simulink model "SISO_Simulation"  (R2020b)
settings: Solver=VariableStepAuto  StartTime=0.0  StopTime=10.0  RelTol=1e-3
PreLoadFcn:
  | loadSystemVariables
values from neighbouring files (symbols this model uses):
  Jl = 6.01e-5    (= 6.01e-05)    [loadSystemVariables.m]
  Jm = 996e-6    (= 0.000996)    [loadSystemVariables.m]
  Kb = (1/1000)*9.5493    (= 0.0095493)    [loadSystemVariables.m]
  Kf = 1    [loadSystemVariables.m]
  Kk = 1e4    (= 10000)    [loadSystemVariables.m]
  Km = 0.5    [loadSystemVariables.m]
  Kt = 18.16e-3    (= 0.01816)    [loadSystemVariables.m]
  Kv = 1000    [loadSystemVariables.m]
  L = series(P,G)    [SISO_phi.m]    (also in SISO_x.m; basicSISO_phi.m; basicSISO_x.m; basicSISO_y.m)
  R = 0.256    [loadSystemVariables.m]
libraries: uavalgslib x1
settings Model: Creator=Iftah  LastModifiedBy=Iftah

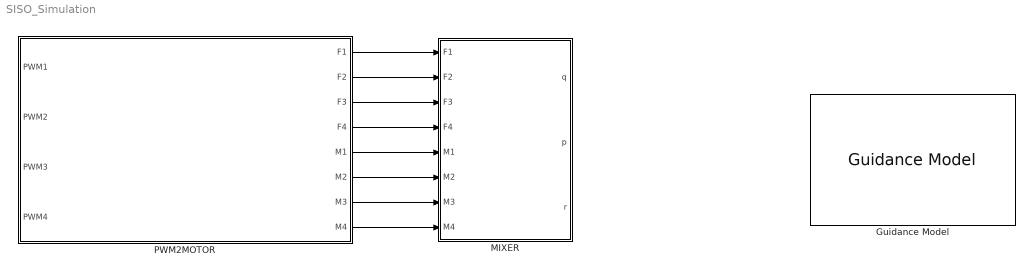
== system SISO_Simulation ==
  Guidance Model : uavalgslib/Guidance Model  ModelType=MultirotorGuidance  SpecifiedDataType=double  SimulateUsing=Interpreted execution  InitialWorldPositionMultirotor=[0; 0; 0]  InitialWorldVelocityMultirotor=[0; 0; 0]  InitialEulerZYXMultirotor=[0; 0; 0]  InitialBodyAngularRateRPYMultirotor=[0; 0; 0]  InitialThrustMultirotor=0  InitialNorthFixedWing=0  InitialEastFixedWing=0  InitialHeightFixedWing=0  InitialAirSpeedFixedWing=0  InitialHeadingAngleFixedWing=0  InitialFlightPathAngleFixedWing=0  InitialRollAngleFixedWing=0  InitialRollAngleRateFixedWing=0  PDRollMultirotor=[3402.97,116.67]  PDPitchMultirotor=[3402.97, 116.67]  PYawRateMultirotor=1950  PThrustMultirotor=3900  MassMultirotor=0.1  PHeightFixedWing=3.9  PHeadingAngleFixedWing=3.9  PFlightPathAngleFixedWing=39  PDRollFixedWing=[3402.97, 116.67]  PAirSpeedFixedWing=1  FlightPathAngleLimitsFixedWing=[-pi/2, pi/2]  StateBusName='MultirotorGuidanceStateBus'  ControlBusName='MultirotorGuidanceControlBus'  EnvironmentBusName='MultirotorGuidanceEnvironmentBus'  DataType=double
      settings: SourceProductBaseCode=UV
  MIXER : Subsystem
  PWM2MOTOR : Subsystem
  wires:
  PWM2MOTOR/1(F1) -> MIXER/1(F1)
  PWM2MOTOR/2(F2) -> MIXER/2(F2)
  PWM2MOTOR/3(F3) -> MIXER/3(F3)
  PWM2MOTOR/4(F4) -> MIXER/4(F4)
  PWM2MOTOR/5(M1) -> MIXER/5(M1)
  PWM2MOTOR/6(M2) -> MIXER/6(M2)
  PWM2MOTOR/7(M3) -> MIXER/7(M3)
  PWM2MOTOR/8(M4) -> MIXER/8(M4)

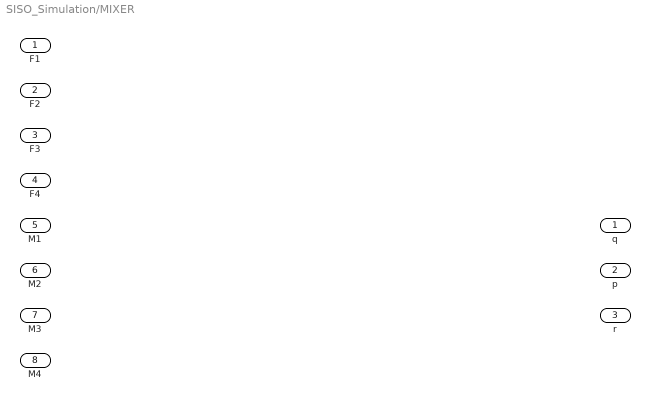
== system SISO_Simulation/MIXER ==
  F1 : Inport
  F2 : Inport  Port=2
  F3 : Inport  Port=3
  F4 : Inport  Port=4
  M1 : Inport  Port=5
  M2 : Inport  Port=6
  M3 : Inport  Port=7
  M4 : Inport  Port=8
  q : Outport
  p : Outport  Port=2
  r : Outport  Port=3

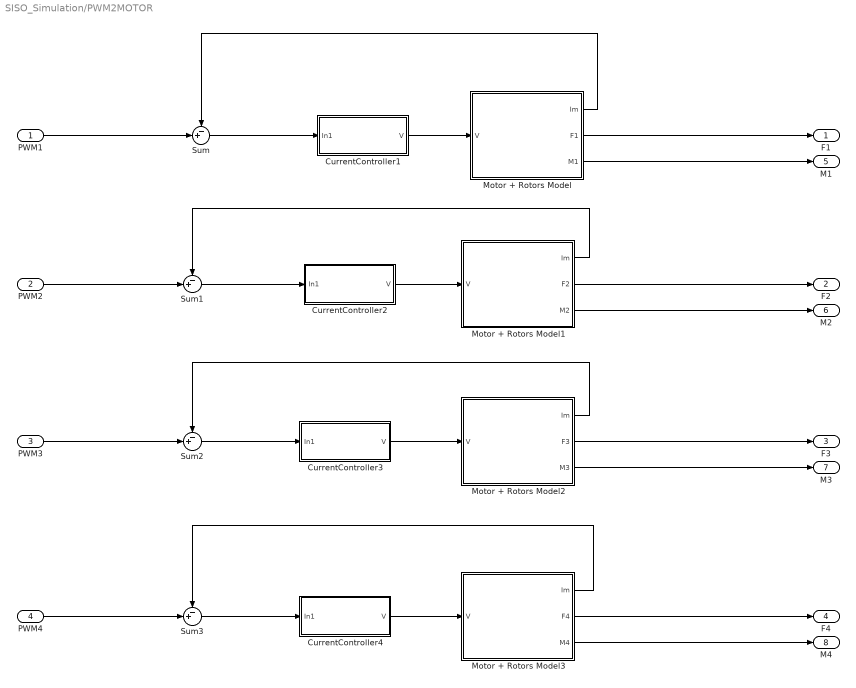
== system SISO_Simulation/PWM2MOTOR ==
  PWM1 : Inport
  PWM2 : Inport  Port=2
  PWM3 : Inport  Port=3
  PWM4 : Inport  Port=4
  CurrentController1 : Subsystem
  CurrentController2 : Subsystem
  CurrentController3 : Subsystem
  CurrentController4 : Subsystem
  Motor + Rotors Model : Subsystem
  Motor + Rotors Model1 : Subsystem
  Motor + Rotors Model2 : Subsystem
  Motor + Rotors Model3 : Subsystem
  Sum{,1..3} (4 alike) : Sum  Inputs=-+|
  F1 : Outport
  F2 : Outport  Port=2
  F3 : Outport  Port=3
  F4 : Outport  Port=4
  M1 : Outport  Port=5
  M2 : Outport  Port=6
  M3 : Outport  Port=7
  M4 : Outport  Port=8
  wires:
  Motor + Rotors Model/2(F1) -> F1/1
  Motor + Rotors Model/1(Im) -> Sum/1
  Motor + Rotors Model3/1(Im) -> Sum3/1
  Motor + Rotors Model1/3(M2) -> M2/1
  CurrentController3/1(V) -> Motor + Rotors Model2/1(V)
  Motor + Rotors Model1/2(F2) -> F2/1
  PWM1/1 -> Sum/2
  CurrentController1/1(V) -> Motor + Rotors Model/1(V)
  PWM3/1 -> Sum2/2
  Sum2/1 -> CurrentController3/1(In1)
  Motor + Rotors Model2/1(Im) -> Sum2/1
  Motor + Rotors Model3/2(F4) -> F4/1
  Sum/1 -> CurrentController1/1(In1)
  Motor + Rotors Model2/2(F3) -> F3/1
  Motor + Rotors Model/3(M1) -> M1/1
  CurrentController2/1(V) -> Motor + Rotors Model1/1(V)
  PWM2/1 -> Sum1/2
  Motor + Rotors Model3/3(M4) -> M4/1
  CurrentController4/1(V) -> Motor + Rotors Model3/1(V)
  Sum3/1 -> CurrentController4/1(In1)
  PWM4/1 -> Sum3/2
  Motor + Rotors Model2/3(M3) -> M3/1
  Sum1/1 -> CurrentController2/1(In1)
  Motor + Rotors Model1/1(Im) -> Sum1/1

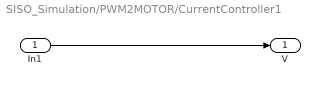
== system SISO_Simulation/PWM2MOTOR/CurrentController1 ==
  In1 : Inport
  V : Outport
  wires:
  In1/1 -> V/1

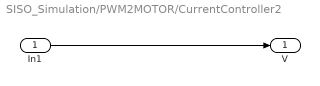
== system SISO_Simulation/PWM2MOTOR/CurrentController2 ==
  In1 : Inport
  V : Outport
  wires:
  In1/1 -> V/1

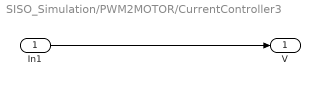
== system SISO_Simulation/PWM2MOTOR/CurrentController3 ==
  In1 : Inport
  V : Outport
  wires:
  In1/1 -> V/1

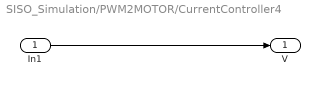
== system SISO_Simulation/PWM2MOTOR/CurrentController4 ==
  In1 : Inport
  V : Outport
  wires:
  In1/1 -> V/1

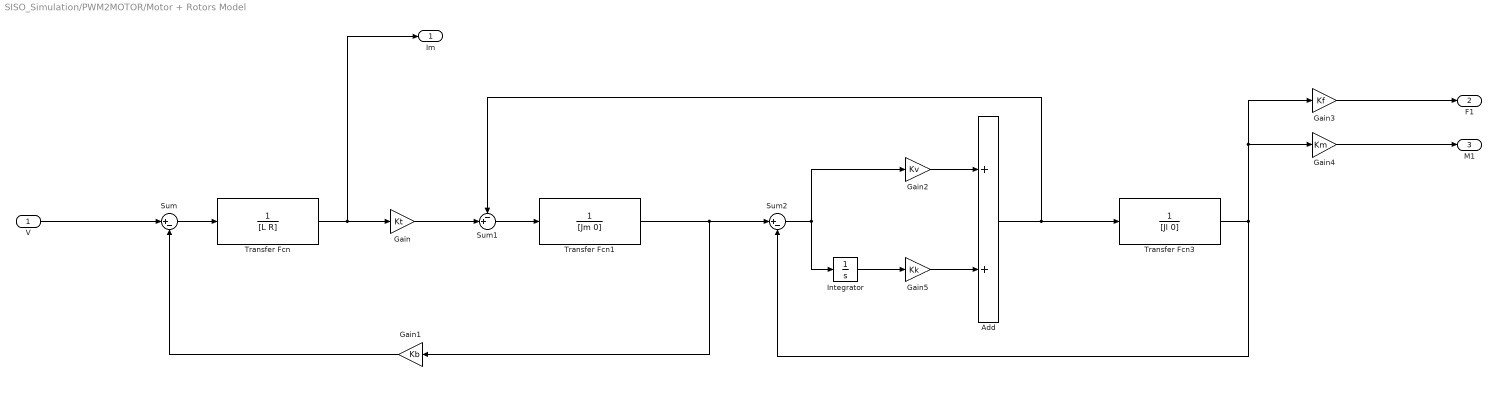
== system SISO_Simulation/PWM2MOTOR/Motor + Rotors Model ==
  V : Inport
  Add : Sum
  Gain : Gain  Gain=Kt
  Gain1 : Gain  Gain=Kb
  Gain2 : Gain  Gain=Kv
  Gain3 : Gain  Gain=Kf
  Gain4 : Gain  Gain=Km
  Gain5 : Gain  Gain=Kk
  Integrator : Integrator
  Sum : Sum  Inputs=|+-
  Sum1 : Sum  Inputs=-+|
  Sum2 : Sum  Inputs=|+-
  Transfer Fcn : TransferFcn  Denominator=[L R]
  Transfer Fcn1 : TransferFcn  Denominator=[Jm 0]
  Transfer Fcn3 : TransferFcn  Denominator=[Jl 0]
  Im : Outport
  F1 : Outport  Port=2
  M1 : Outport  Port=3
  wires:
  V/1 -> Sum/1
  Transfer Fcn/1 -> Im/1, Gain/1
  Transfer Fcn1/1 -> Sum2/1, Gain1/1
  Sum/1 -> Transfer Fcn/1
  Gain1/1 -> Sum/2
  Gain/1 -> Sum1/2
  Sum1/1 -> Transfer Fcn1/1
  Sum2/1 -> Integrator/1, Gain2/1
  Gain2/1 -> Add/1
  Gain5/1 -> Add/2
  Add/1 -> Transfer Fcn3/1, Sum1/1
  Transfer Fcn3/1 -> Gain3/1, Gain4/1, Sum2/2
  Gain3/1 -> F1/1
  Gain4/1 -> M1/1
  Integrator/1 -> Gain5/1

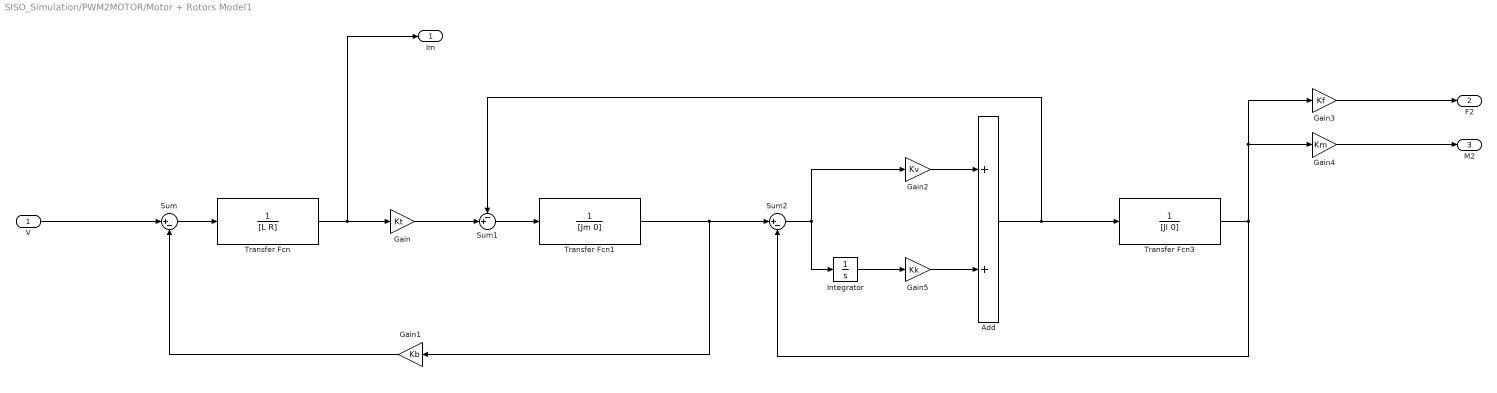
== system SISO_Simulation/PWM2MOTOR/Motor + Rotors Model1 ==
  V : Inport
  Add : Sum
  Gain : Gain  Gain=Kt
  Gain1 : Gain  Gain=Kb
  Gain2 : Gain  Gain=Kv
  Gain3 : Gain  Gain=Kf
  Gain4 : Gain  Gain=Km
  Gain5 : Gain  Gain=Kk
  Integrator : Integrator
  Sum : Sum  Inputs=|+-
  Sum1 : Sum  Inputs=-+|
  Sum2 : Sum  Inputs=|+-
  Transfer Fcn : TransferFcn  Denominator=[L R]
  Transfer Fcn1 : TransferFcn  Denominator=[Jm 0]
  Transfer Fcn3 : TransferFcn  Denominator=[Jl 0]
  Im : Outport
  F2 : Outport  Port=2
  M2 : Outport  Port=3
  wires:
  V/1 -> Sum/1
  Transfer Fcn/1 -> Im/1, Gain/1
  Transfer Fcn1/1 -> Sum2/1, Gain1/1
  Sum/1 -> Transfer Fcn/1
  Gain1/1 -> Sum/2
  Gain/1 -> Sum1/2
  Sum1/1 -> Transfer Fcn1/1
  Sum2/1 -> Integrator/1, Gain2/1
  Gain2/1 -> Add/1
  Gain5/1 -> Add/2
  Add/1 -> Transfer Fcn3/1, Sum1/1
  Transfer Fcn3/1 -> Gain3/1, Gain4/1, Sum2/2
  Gain3/1 -> F2/1
  Gain4/1 -> M2/1
  Integrator/1 -> Gain5/1

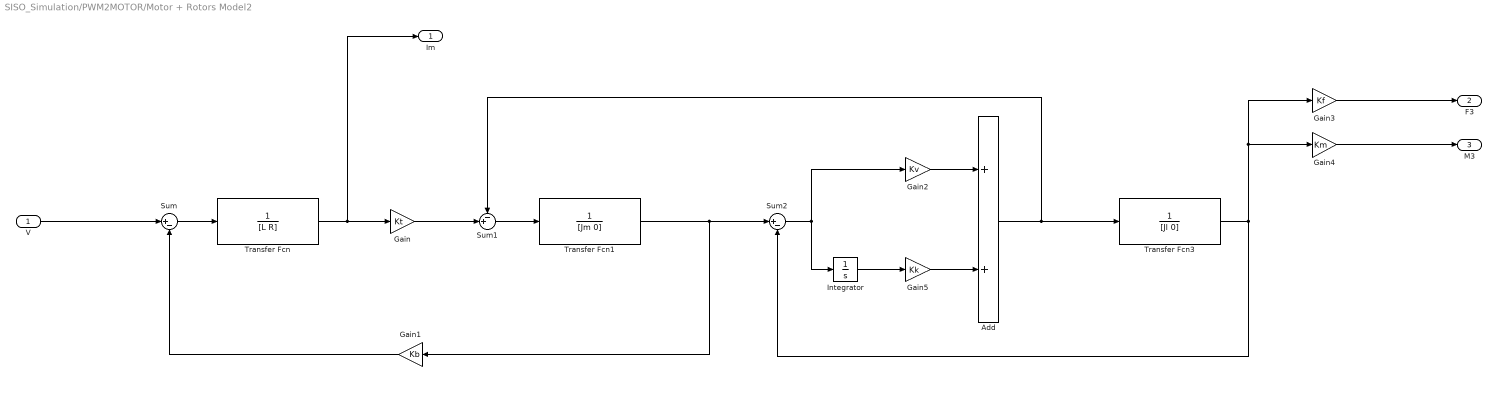
== system SISO_Simulation/PWM2MOTOR/Motor + Rotors Model2 ==
  V : Inport
  Add : Sum
  Gain : Gain  Gain=Kt
  Gain1 : Gain  Gain=Kb
  Gain2 : Gain  Gain=Kv
  Gain3 : Gain  Gain=Kf
  Gain4 : Gain  Gain=Km
  Gain5 : Gain  Gain=Kk
  Integrator : Integrator
  Sum : Sum  Inputs=|+-
  Sum1 : Sum  Inputs=-+|
  Sum2 : Sum  Inputs=|+-
  Transfer Fcn : TransferFcn  Denominator=[L R]
  Transfer Fcn1 : TransferFcn  Denominator=[Jm 0]
  Transfer Fcn3 : TransferFcn  Denominator=[Jl 0]
  Im : Outport
  F3 : Outport  Port=2
  M3 : Outport  Port=3
  wires:
  V/1 -> Sum/1
  Transfer Fcn/1 -> Im/1, Gain/1
  Transfer Fcn1/1 -> Sum2/1, Gain1/1
  Sum/1 -> Transfer Fcn/1
  Gain1/1 -> Sum/2
  Gain/1 -> Sum1/2
  Sum1/1 -> Transfer Fcn1/1
  Sum2/1 -> Integrator/1, Gain2/1
  Gain2/1 -> Add/1
  Gain5/1 -> Add/2
  Add/1 -> Transfer Fcn3/1, Sum1/1
  Transfer Fcn3/1 -> Gain3/1, Gain4/1, Sum2/2
  Gain3/1 -> F3/1
  Gain4/1 -> M3/1
  Integrator/1 -> Gain5/1

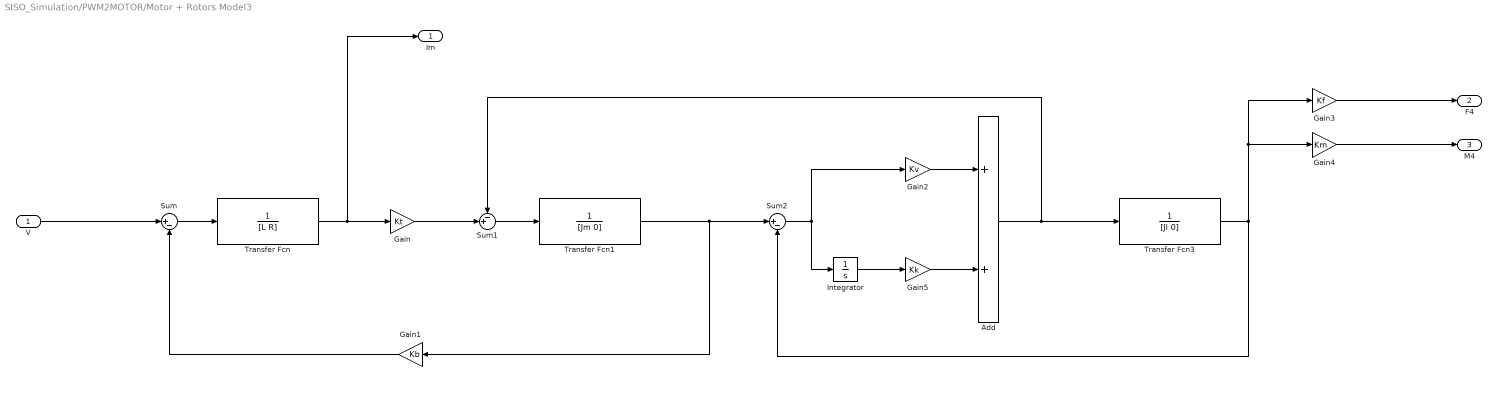
== system SISO_Simulation/PWM2MOTOR/Motor + Rotors Model3 ==
  V : Inport
  Add : Sum
  Gain : Gain  Gain=Kt
  Gain1 : Gain  Gain=Kb
  Gain2 : Gain  Gain=Kv
  Gain3 : Gain  Gain=Kf
  Gain4 : Gain  Gain=Km
  Gain5 : Gain  Gain=Kk
  Integrator : Integrator
  Sum : Sum  Inputs=|+-
  Sum1 : Sum  Inputs=-+|
  Sum2 : Sum  Inputs=|+-
  Transfer Fcn : TransferFcn  Denominator=[L R]
  Transfer Fcn1 : TransferFcn  Denominator=[Jm 0]
  Transfer Fcn3 : TransferFcn  Denominator=[Jl 0]
  Im : Outport
  F4 : Outport  Port=2
  M4 : Outport  Port=3
  wires:
  V/1 -> Sum/1
  Transfer Fcn/1 -> Im/1, Gain/1
  Transfer Fcn1/1 -> Sum2/1, Gain1/1
  Sum/1 -> Transfer Fcn/1
  Gain1/1 -> Sum/2
  Gain/1 -> Sum1/2
  Sum1/1 -> Transfer Fcn1/1
  Sum2/1 -> Integrator/1, Gain2/1
  Gain2/1 -> Add/1
  Gain5/1 -> Add/2
  Add/1 -> Transfer Fcn3/1, Sum1/1
  Transfer Fcn3/1 -> Gain3/1, Gain4/1, Sum2/2
  Gain3/1 -> F4/1
  Gain4/1 -> M4/1
  Integrator/1 -> Gain5/1
